simulink model "TI_BQ76952"  (R2026a)
settings: Solver=FixedStepDiscrete  StopTime=t_sim_end  FixedStep=T_s
values from neighbouring files (symbols this model uses):
  Cell5_Select = zeros(num_cells, 1)    [TI_BQ76952_params.m]
  Cell_Base_V = 3.7    [TI_BQ76952_params.m]
  N_COV_Delay_Ticks = round(t_COV_Delay / T_s)    [TI_BQ76952_params.m]
  N_CUV_Delay_Ticks = round(t_CUV_Delay / T_s)    [TI_BQ76952_params.m]
  num_cells = 14    [TI_BQ76952_params.m]
  t_Phase1 = 1.0    (= 1)    [TI_BQ76952_params.m]
  t_Phase2 = 2.0    (= 2)    [TI_BQ76952_params.m]
  t_Phase3 = 3.0    (= 3)    [TI_BQ76952_params.m]
  T_s = 1e-3    (= 0.001)    [TI_BQ76952_params.m]
  V_Cell5_Phase1 = 4.3    [TI_BQ76952_params.m]
  V_Cell5_Phase2 = 4.2    [TI_BQ76952_params.m]
  V_Cell5_Phase3 = 4.1    [TI_BQ76952_params.m]
  V_COV_Hyst = 0.100    (= 0.1)    [TI_BQ76952_params.m]
  V_COV_Thresh = 4.25    [TI_BQ76952_params.m]
  V_CUV_Hyst = 0.100    (= 0.1)    [TI_BQ76952_params.m]
  V_CUV_Thresh = 2.75    [TI_BQ76952_params.m]
settings Model: Creator=Razvan  LastModifiedBy=Razvan

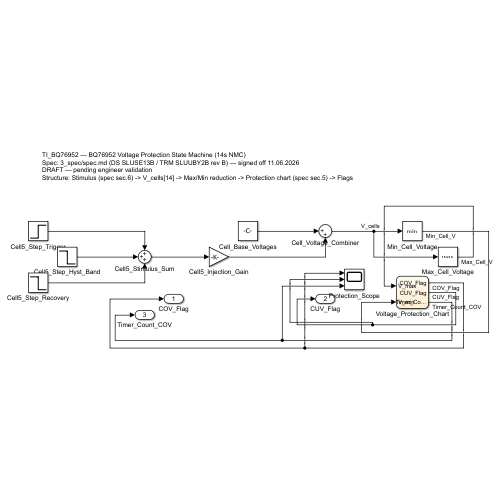
[thumbnail: Simulink's stored preview of the top-level diagram]
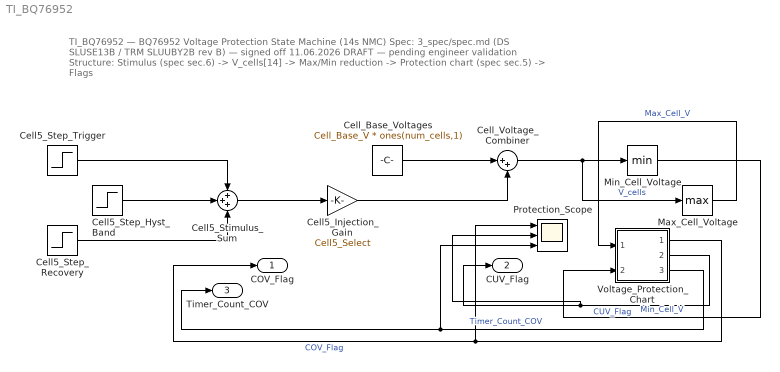
== system TI_BQ76952 ==
  note: TI_BQ76952 — BQ76952 Voltage Protection State Machine (14s NMC)
      | Spec: 3_spec/spec.md (DS SLUSE13B / TRM SLUUBY2B rev B) — signed off 11.06.2026
      | DRAFT — pending engineer validation
      | Structure: Stimulus (spec sec.6) -> V_cells[14] -> Max/Min reduction -> Protection chart (spec sec.5) -> Flags
  Cell5_Injection_Gain : Gain  Description=spec sec.6: routes scalar stimulus onto cell #5 only (Cell5_Select vector, Stim_Cell_Idx = 5)  Gain=Cell5_Select
  Cell5_Step_Hyst_Band : Step  Description=spec sec.6: cell #5 drops to 4.2 V at t = 2.0 s (inside hysteresis band)  Time=t_Phase2  FinalValue=V_Cell5_Phase2 - V_Cell5_Phase1  SampleTime=T_s
  Cell5_Step_Recovery : Step  Description=spec sec.6: cell #5 drops to 4.1 V at t = 3.0 s (full recovery)  Time=t_Phase3  FinalValue=V_Cell5_Phase3 - V_Cell5_Phase2  SampleTime=T_s
  Cell5_Step_Trigger : Step  Description=spec sec.6: cell #5 steps to 4.3 V at t = 1.0 s (triggering condition)  Time=t_Phase1  FinalValue=V_Cell5_Phase1 - Cell_Base_V  SampleTime=T_s
  Cell5_Stimulus_Sum : Sum  Description=spec sec.6: composes the cell #5 voltage deviation profile from the three steps  Inputs=+++
  Cell_Base_Voltages : Constant  Description=spec sec.6: all 14 cells steady at 3.7 V (Cell_Base_V, num_cells per spec sec.3)  Value=Cell_Base_V * ones(num_cells,1)  SampleTime=T_s
  Cell_Voltage_Combiner : Sum  Description=spec sec.6: V_cells[14] = base 3.7 V vector + cell #5 stimulus deviation  Inputs=|++
  Max_Cell_Voltage : MinMax  Description=config fixed architecture: V_cells -> Max_Cell_V reduction, feeds COV machine (spec sec.5: ANY cell >= threshold)  Function=max
  Min_Cell_Voltage : MinMax  Description=config fixed architecture: V_cells -> Min_Cell_V reduction, feeds CUV machine (spec sec.5)
  Protection_Scope : Scope  NumInputPorts=3
      settings: Description=spec sec.6 outputs: COV_Flag, CUV_Flag, Timer_Count_COV
  Voltage_Protection_Chart : Stateflow chart  Description=spec sec.5: COV/CUV protection state machines with delay timers (spec sec.3) and recovery hysteresis (spec sec.4)  TreatAsAtomicUnit=on
  COV_Flag : Outport  Description=spec sec.6 output: COV_Flag
  CUV_Flag : Outport  Description=spec sec.6 output: CUV_Flag  Port=2
  Timer_Count_COV : Outport  Description=spec sec.6 output: Timer_Count_COV (AC2)  Port=3
  wires:
  Cell5_Step_Trigger/1 -> Cell5_Stimulus_Sum/1
  Cell5_Step_Hyst_Band/1 -> Cell5_Stimulus_Sum/2
  Cell5_Step_Recovery/1 -> Cell5_Stimulus_Sum/3
  Cell5_Stimulus_Sum/1 -> Cell5_Injection_Gain/1
  Cell_Base_Voltages/1 -> Cell_Voltage_Combiner/1
  Cell5_Injection_Gain/1 -> Cell_Voltage_Combiner/2
  Cell_Voltage_Combiner/1 -> Min_Cell_Voltage/1, Max_Cell_Voltage/1  "V_cells"
  Max_Cell_Voltage/1 -> Voltage_Protection_Chart/1(V_max)  "Max_Cell_V"
  Min_Cell_Voltage/1 -> Voltage_Protection_Chart/2(V_min)  "Min_Cell_V"
  Voltage_Protection_Chart/1(COV_Flag) -> COV_Flag/1, Protection_Scope/1  "COV_Flag"
  Voltage_Protection_Chart/2(CUV_Flag) -> Protection_Scope/2, CUV_Flag/1  "CUV_Flag"
  Voltage_Protection_Chart/3(Timer_Count_COV) -> Protection_Scope/3, Timer_Count_COV/1  "Timer_Count_COV"

== stateflow chart TI_BQ76952/Voltage_Protection_Chart ==
  settings: updateMethod=DISCRETE  sampleTime=T_s
  state CUV_Machine [parallel]
    settings: executionOrder=1
    state CUV_Normal
      en:
      CUV_Flag = 0;
      Timer_Count_CUV = 0;
    state CUV_Delay_Count
      du:
      Timer_Count_CUV = Timer_Count_CUV + 1;
    state CUV_Faulted
      en:
      CUV_Flag = 1;
    (default) -> CUV_Normal
    CUV_Faulted -> CUV_Normal : [V_min >= V_CUV_Thresh + V_CUV_Hyst]
    CUV_Delay_Count -> CUV_Normal [order 2] : [V_min > V_CUV_Thresh]
    CUV_Normal -> CUV_Delay_Count : [V_min <= V_CUV_Thresh]
    CUV_Delay_Count -> CUV_Faulted [order 1] : [Timer_Count_CUV >= N_CUV_Delay_Ticks]
  state COV_Machine [parallel]
    settings: executionOrder=2
    state COV_Normal
      en:
      COV_Flag = 0;
      Timer_Count_COV = 0;
    state COV_Delay_Count
      du:
      Timer_Count_COV = Timer_Count_COV + 1;
    state COV_Faulted
      en:
      COV_Flag = 1;
    (default) -> COV_Normal
    COV_Faulted -> COV_Normal : [V_max <= V_COV_Thresh - V_COV_Hyst]
    COV_Normal -> COV_Delay_Count : [V_max >= V_COV_Thresh]
    COV_Delay_Count -> COV_Normal [order 2] : [V_max < V_COV_Thresh]
    COV_Delay_Count -> COV_Faulted [order 1] : [Timer_Count_COV >= N_COV_Delay_Ticks]
  data: V_max input double; V_min input double; COV_Flag output double; CUV_Flag output double; Timer_Count_COV output double; Timer_Count_CUV local double; V_COV_Thresh parameter double; V_COV_Hyst parameter double; N_COV_Delay_Ticks parameter double; V_CUV_Thresh parameter double; V_CUV_Hyst parameter double; N_CUV_Delay_Ticks parameter double
